simulink model "kurtosis"  (R2012b)
settings: Solver=ode45  StartTime=0.0  StopTime=3171  RelTol=1e-3
libraries: xbsIndex_r4 x3174, casper_library_flow_control x64, casper_library_misc x1, simulink_xsg_bridge x1
(part 3 of 24)

== system kurtosis/kurtosis/kurtosis_origin_moments_2 ==
  sync_in : Inport
  x_in : Inport  Port=2
  abs_x_sq : Subsystem
  abs_x_sq_del : xbsIndex_r4/Delay  rst=off  infoeditControl=Selection of Reset will increase slice count due to use of real FFs and instead of SRLs  en=off  latency=5  dbl_ovrd=off  reg_retiming=off  block_type=delay
  c_to_ri_xin : Subsystem
  cplx_sq : Subsystem
  ri_to_c_x_3rd : Subsystem
  square_real : xbsIndex_r4/Mult  precision=Full  arith_type="Signed  (2's comp)"  n_bits=36  bin_pt=34  quantization=Truncate  overflow=Wrap  en=off  latency=5  dbl_ovrd=off  use_behavioral_HDL=off  opt=Speed  use_embedded=on  optimum_pipeline=off  pipeline=on  use_rpm=on  placement_style=Triangular  block_type=mult
  sync_delay : xbsIndex_r4/Delay  rst=off  infoeditControl=Selection of Reset will increase slice count due to use of real FFs and instead of SRLs  en=off  latency=10  dbl_ovrd=off  reg_retiming=off  block_type=delay
  third_power_im : xbsIndex_r4/Mult  precision=Full  arith_type="Signed  (2's comp)"  n_bits=36  bin_pt=34  quantization=Truncate  overflow=Wrap  en=off  latency=5  dbl_ovrd=off  use_behavioral_HDL=off  opt=Speed  use_embedded=on  optimum_pipeline=off  pipeline=on  use_rpm=on  placement_style=Triangular  block_type=mult
  third_power_re : xbsIndex_r4/Mult  precision=Full  arith_type="Signed  (2's comp)"  n_bits=36  bin_pt=34  quantization=Truncate  overflow=Wrap  en=off  latency=5  dbl_ovrd=off  use_behavioral_HDL=off  opt=Speed  use_embedded=on  optimum_pipeline=off  pipeline=on  use_rpm=on  placement_style=Triangular  block_type=mult
  x_delay : xbsIndex_r4/Delay  rst=off  infoeditControl=Selection of Reset will increase slice count due to use of real FFs and instead of SRLs  en=off  latency=10  dbl_ovrd=off  reg_retiming=off  block_type=delay
  x_im_del : xbsIndex_r4/Delay  rst=off  infoeditControl=Selection of Reset will increase slice count due to use of real FFs and instead of SRLs  en=off  latency=5  dbl_ovrd=off  reg_retiming=off  block_type=delay
  x_re_del : xbsIndex_r4/Delay  rst=off  infoeditControl=Selection of Reset will increase slice count due to use of real FFs and instead of SRLs  en=off  latency=5  dbl_ovrd=off  reg_retiming=off  block_type=delay
  x_sq_del : xbsIndex_r4/Delay  rst=off  infoeditControl=Selection of Reset will increase slice count due to use of real FFs and instead of SRLs  en=off  latency=4  dbl_ovrd=off  reg_retiming=off  block_type=delay
  sync_out : Outport
  x : Outport  Port=2
  x^2 : Outport  Port=3
  |x|^2 : Outport  Port=4
  |x|^4 : Outport  Port=5
  x|x|^2 : Outport  Port=6
  wires:
  x_in/1 -> c_to_ri_xin/1(c), abs_x_sq/1(c), cplx_sq/2(b), cplx_sq/1(a), x_delay/1
  abs_x_sq/1(power) -> third_power_im/2, third_power_re/2, square_real/2, square_real/1, abs_x_sq_del/1
  ri_to_c_x_3rd/1(c) -> x|x|^2/1
  third_power_im/1 -> ri_to_c_x_3rd/2(im)
  third_power_re/1 -> ri_to_c_x_3rd/1(re)
  x_im_del/1 -> third_power_im/1
  x_re_del/1 -> third_power_re/1
  c_to_ri_xin/2(im) -> x_im_del/1
  c_to_ri_xin/1(re) -> x_re_del/1
  square_real/1 -> |x|^4/1
  abs_x_sq_del/1 -> |x|^2/1
  x_sq_del/1 -> x^2/1
  cplx_sq/1(c) -> x_sq_del/1
  x_delay/1 -> x/1
  sync_delay/1 -> sync_out/1
  sync_in/1 -> sync_delay/1

== system kurtosis/kurtosis/kurtosis_origin_moments_3 ==
  sync_in : Inport
  x_in : Inport  Port=2
  abs_x_sq : Subsystem
  abs_x_sq_del : xbsIndex_r4/Delay  rst=off  infoeditControl=Selection of Reset will increase slice count due to use of real FFs and instead of SRLs  en=off  latency=5  dbl_ovrd=off  reg_retiming=off  block_type=delay
  c_to_ri_xin : Subsystem
  cplx_sq : Subsystem
  ri_to_c_x_3rd : Subsystem
  square_real : xbsIndex_r4/Mult  precision=Full  arith_type="Signed  (2's comp)"  n_bits=36  bin_pt=34  quantization=Truncate  overflow=Wrap  en=off  latency=5  dbl_ovrd=off  use_behavioral_HDL=off  opt=Speed  use_embedded=on  optimum_pipeline=off  pipeline=on  use_rpm=on  placement_style=Triangular  block_type=mult
  sync_delay : xbsIndex_r4/Delay  rst=off  infoeditControl=Selection of Reset will increase slice count due to use of real FFs and instead of SRLs  en=off  latency=10  dbl_ovrd=off  reg_retiming=off  block_type=delay
  third_power_im : xbsIndex_r4/Mult  precision=Full  arith_type="Signed  (2's comp)"  n_bits=36  bin_pt=34  quantization=Truncate  overflow=Wrap  en=off  latency=5  dbl_ovrd=off  use_behavioral_HDL=off  opt=Speed  use_embedded=on  optimum_pipeline=off  pipeline=on  use_rpm=on  placement_style=Triangular  block_type=mult
  third_power_re : xbsIndex_r4/Mult  precision=Full  arith_type="Signed  (2's comp)"  n_bits=36  bin_pt=34  quantization=Truncate  overflow=Wrap  en=off  latency=5  dbl_ovrd=off  use_behavioral_HDL=off  opt=Speed  use_embedded=on  optimum_pipeline=off  pipeline=on  use_rpm=on  placement_style=Triangular  block_type=mult
  x_delay : xbsIndex_r4/Delay  rst=off  infoeditControl=Selection of Reset will increase slice count due to use of real FFs and instead of SRLs  en=off  latency=10  dbl_ovrd=off  reg_retiming=off  block_type=delay
  x_im_del : xbsIndex_r4/Delay  rst=off  infoeditControl=Selection of Reset will increase slice count due to use of real FFs and instead of SRLs  en=off  latency=5  dbl_ovrd=off  reg_retiming=off  block_type=delay
  x_re_del : xbsIndex_r4/Delay  rst=off  infoeditControl=Selection of Reset will increase slice count due to use of real FFs and instead of SRLs  en=off  latency=5  dbl_ovrd=off  reg_retiming=off  block_type=delay
  x_sq_del : xbsIndex_r4/Delay  rst=off  infoeditControl=Selection of Reset will increase slice count due to use of real FFs and instead of SRLs  en=off  latency=4  dbl_ovrd=off  reg_retiming=off  block_type=delay
  sync_out : Outport
  x : Outport  Port=2
  x^2 : Outport  Port=3
  |x|^2 : Outport  Port=4
  |x|^4 : Outport  Port=5
  x|x|^2 : Outport  Port=6
  wires:
  x_in/1 -> c_to_ri_xin/1(c), abs_x_sq/1(c), cplx_sq/2(b), cplx_sq/1(a), x_delay/1
  abs_x_sq/1(power) -> third_power_im/2, third_power_re/2, square_real/2, square_real/1, abs_x_sq_del/1
  ri_to_c_x_3rd/1(c) -> x|x|^2/1
  third_power_im/1 -> ri_to_c_x_3rd/2(im)
  third_power_re/1 -> ri_to_c_x_3rd/1(re)
  x_im_del/1 -> third_power_im/1
  x_re_del/1 -> third_power_re/1
  c_to_ri_xin/2(im) -> x_im_del/1
  c_to_ri_xin/1(re) -> x_re_del/1
  square_real/1 -> |x|^4/1
  abs_x_sq_del/1 -> |x|^2/1
  x_sq_del/1 -> x^2/1
  cplx_sq/1(c) -> x_sq_del/1
  x_delay/1 -> x/1
  sync_delay/1 -> sync_out/1
  sync_in/1 -> sync_delay/1

== system kurtosis/kurtosis/kurtosis_origin_moments_4 ==
  sync_in : Inport
  x_in : Inport  Port=2
  abs_x_sq : Subsystem
  abs_x_sq_del : xbsIndex_r4/Delay  rst=off  infoeditControl=Selection of Reset will increase slice count due to use of real FFs and instead of SRLs  en=off  latency=5  dbl_ovrd=off  reg_retiming=off  block_type=delay
  c_to_ri_xin : Subsystem
  cplx_sq : Subsystem
  ri_to_c_x_3rd : Subsystem
  square_real : xbsIndex_r4/Mult  precision=Full  arith_type="Signed  (2's comp)"  n_bits=36  bin_pt=34  quantization=Truncate  overflow=Wrap  en=off  latency=5  dbl_ovrd=off  use_behavioral_HDL=off  opt=Speed  use_embedded=on  optimum_pipeline=off  pipeline=on  use_rpm=on  placement_style=Triangular  block_type=mult
  sync_delay : xbsIndex_r4/Delay  rst=off  infoeditControl=Selection of Reset will increase slice count due to use of real FFs and instead of SRLs  en=off  latency=10  dbl_ovrd=off  reg_retiming=off  block_type=delay
  third_power_im : xbsIndex_r4/Mult  precision=Full  arith_type="Signed  (2's comp)"  n_bits=36  bin_pt=34  quantization=Truncate  overflow=Wrap  en=off  latency=5  dbl_ovrd=off  use_behavioral_HDL=off  opt=Speed  use_embedded=on  optimum_pipeline=off  pipeline=on  use_rpm=on  placement_style=Triangular  block_type=mult
  third_power_re : xbsIndex_r4/Mult  precision=Full  arith_type="Signed  (2's comp)"  n_bits=36  bin_pt=34  quantization=Truncate  overflow=Wrap  en=off  latency=5  dbl_ovrd=off  use_behavioral_HDL=off  opt=Speed  use_embedded=on  optimum_pipeline=off  pipeline=on  use_rpm=on  placement_style=Triangular  block_type=mult
  x_delay : xbsIndex_r4/Delay  rst=off  infoeditControl=Selection of Reset will increase slice count due to use of real FFs and instead of SRLs  en=off  latency=10  dbl_ovrd=off  reg_retiming=off  block_type=delay
  x_im_del : xbsIndex_r4/Delay  rst=off  infoeditControl=Selection of Reset will increase slice count due to use of real FFs and instead of SRLs  en=off  latency=5  dbl_ovrd=off  reg_retiming=off  block_type=delay
  x_re_del : xbsIndex_r4/Delay  rst=off  infoeditControl=Selection of Reset will increase slice count due to use of real FFs and instead of SRLs  en=off  latency=5  dbl_ovrd=off  reg_retiming=off  block_type=delay
  x_sq_del : xbsIndex_r4/Delay  rst=off  infoeditControl=Selection of Reset will increase slice count due to use of real FFs and instead of SRLs  en=off  latency=4  dbl_ovrd=off  reg_retiming=off  block_type=delay
  sync_out : Outport
  x : Outport  Port=2
  x^2 : Outport  Port=3
  |x|^2 : Outport  Port=4
  |x|^4 : Outport  Port=5
  x|x|^2 : Outport  Port=6
  wires:
  x_in/1 -> c_to_ri_xin/1(c), abs_x_sq/1(c), cplx_sq/2(b), cplx_sq/1(a), x_delay/1
  abs_x_sq/1(power) -> third_power_im/2, third_power_re/2, square_real/2, square_real/1, abs_x_sq_del/1
  ri_to_c_x_3rd/1(c) -> x|x|^2/1
  third_power_im/1 -> ri_to_c_x_3rd/2(im)
  third_power_re/1 -> ri_to_c_x_3rd/1(re)
  x_im_del/1 -> third_power_im/1
  x_re_del/1 -> third_power_re/1
  c_to_ri_xin/2(im) -> x_im_del/1
  c_to_ri_xin/1(re) -> x_re_del/1
  square_real/1 -> |x|^4/1
  abs_x_sq_del/1 -> |x|^2/1
  x_sq_del/1 -> x^2/1
  cplx_sq/1(c) -> x_sq_del/1
  x_delay/1 -> x/1
  sync_delay/1 -> sync_out/1
  sync_in/1 -> sync_delay/1

== system kurtosis/kurtosis/kurtosis_origin_moments_5 ==
  sync_in : Inport
  x_in : Inport  Port=2
  abs_x_sq : Subsystem
  abs_x_sq_del : xbsIndex_r4/Delay  rst=off  infoeditControl=Selection of Reset will increase slice count due to use of real FFs and instead of SRLs  en=off  latency=5  dbl_ovrd=off  reg_retiming=off  block_type=delay
  c_to_ri_xin : Subsystem
  cplx_sq : Subsystem
  ri_to_c_x_3rd : Subsystem
  square_real : xbsIndex_r4/Mult  precision=Full  arith_type="Signed  (2's comp)"  n_bits=36  bin_pt=34  quantization=Truncate  overflow=Wrap  en=off  latency=5  dbl_ovrd=off  use_behavioral_HDL=off  opt=Speed  use_embedded=on  optimum_pipeline=off  pipeline=on  use_rpm=on  placement_style=Triangular  block_type=mult
  sync_delay : xbsIndex_r4/Delay  rst=off  infoeditControl=Selection of Reset will increase slice count due to use of real FFs and instead of SRLs  en=off  latency=10  dbl_ovrd=off  reg_retiming=off  block_type=delay
  third_power_im : xbsIndex_r4/Mult  precision=Full  arith_type="Signed  (2's comp)"  n_bits=36  bin_pt=34  quantization=Truncate  overflow=Wrap  en=off  latency=5  dbl_ovrd=off  use_behavioral_HDL=off  opt=Speed  use_embedded=on  optimum_pipeline=off  pipeline=on  use_rpm=on  placement_style=Triangular  block_type=mult
  third_power_re : xbsIndex_r4/Mult  precision=Full  arith_type="Signed  (2's comp)"  n_bits=36  bin_pt=34  quantization=Truncate  overflow=Wrap  en=off  latency=5  dbl_ovrd=off  use_behavioral_HDL=off  opt=Speed  use_embedded=on  optimum_pipeline=off  pipeline=on  use_rpm=on  placement_style=Triangular  block_type=mult
  x_delay : xbsIndex_r4/Delay  rst=off  infoeditControl=Selection of Reset will increase slice count due to use of real FFs and instead of SRLs  en=off  latency=10  dbl_ovrd=off  reg_retiming=off  block_type=delay
  x_im_del : xbsIndex_r4/Delay  rst=off  infoeditControl=Selection of Reset will increase slice count due to use of real FFs and instead of SRLs  en=off  latency=5  dbl_ovrd=off  reg_retiming=off  block_type=delay
  x_re_del : xbsIndex_r4/Delay  rst=off  infoeditControl=Selection of Reset will increase slice count due to use of real FFs and instead of SRLs  en=off  latency=5  dbl_ovrd=off  reg_retiming=off  block_type=delay
  x_sq_del : xbsIndex_r4/Delay  rst=off  infoeditControl=Selection of Reset will increase slice count due to use of real FFs and instead of SRLs  en=off  latency=4  dbl_ovrd=off  reg_retiming=off  block_type=delay
  sync_out : Outport
  x : Outport  Port=2
  x^2 : Outport  Port=3
  |x|^2 : Outport  Port=4
  |x|^4 : Outport  Port=5
  x|x|^2 : Outport  Port=6
  wires:
  x_in/1 -> c_to_ri_xin/1(c), abs_x_sq/1(c), cplx_sq/2(b), cplx_sq/1(a), x_delay/1
  abs_x_sq/1(power) -> third_power_im/2, third_power_re/2, square_real/2, square_real/1, abs_x_sq_del/1
  ri_to_c_x_3rd/1(c) -> x|x|^2/1
  third_power_im/1 -> ri_to_c_x_3rd/2(im)
  third_power_re/1 -> ri_to_c_x_3rd/1(re)
  x_im_del/1 -> third_power_im/1
  x_re_del/1 -> third_power_re/1
  c_to_ri_xin/2(im) -> x_im_del/1
  c_to_ri_xin/1(re) -> x_re_del/1
  square_real/1 -> |x|^4/1
  abs_x_sq_del/1 -> |x|^2/1
  x_sq_del/1 -> x^2/1
  cplx_sq/1(c) -> x_sq_del/1
  x_delay/1 -> x/1
  sync_delay/1 -> sync_out/1
  sync_in/1 -> sync_delay/1

== system kurtosis/kurtosis/kurtosis_origin_moments_6 ==
  sync_in : Inport
  x_in : Inport  Port=2
  abs_x_sq : Subsystem
  abs_x_sq_del : xbsIndex_r4/Delay  rst=off  infoeditControl=Selection of Reset will increase slice count due to use of real FFs and instead of SRLs  en=off  latency=5  dbl_ovrd=off  reg_retiming=off  block_type=delay
  c_to_ri_xin : Subsystem
  cplx_sq : Subsystem
  ri_to_c_x_3rd : Subsystem
  square_real : xbsIndex_r4/Mult  precision=Full  arith_type="Signed  (2's comp)"  n_bits=36  bin_pt=34  quantization=Truncate  overflow=Wrap  en=off  latency=5  dbl_ovrd=off  use_behavioral_HDL=off  opt=Speed  use_embedded=on  optimum_pipeline=off  pipeline=on  use_rpm=on  placement_style=Triangular  block_type=mult
  sync_delay : xbsIndex_r4/Delay  rst=off  infoeditControl=Selection of Reset will increase slice count due to use of real FFs and instead of SRLs  en=off  latency=10  dbl_ovrd=off  reg_retiming=off  block_type=delay
  third_power_im : xbsIndex_r4/Mult  precision=Full  arith_type="Signed  (2's comp)"  n_bits=36  bin_pt=34  quantization=Truncate  overflow=Wrap  en=off  latency=5  dbl_ovrd=off  use_behavioral_HDL=off  opt=Speed  use_embedded=on  optimum_pipeline=off  pipeline=on  use_rpm=on  placement_style=Triangular  block_type=mult
  third_power_re : xbsIndex_r4/Mult  precision=Full  arith_type="Signed  (2's comp)"  n_bits=36  bin_pt=34  quantization=Truncate  overflow=Wrap  en=off  latency=5  dbl_ovrd=off  use_behavioral_HDL=off  opt=Speed  use_embedded=on  optimum_pipeline=off  pipeline=on  use_rpm=on  placement_style=Triangular  block_type=mult
  x_delay : xbsIndex_r4/Delay  rst=off  infoeditControl=Selection of Reset will increase slice count due to use of real FFs and instead of SRLs  en=off  latency=10  dbl_ovrd=off  reg_retiming=off  block_type=delay
  x_im_del : xbsIndex_r4/Delay  rst=off  infoeditControl=Selection of Reset will increase slice count due to use of real FFs and instead of SRLs  en=off  latency=5  dbl_ovrd=off  reg_retiming=off  block_type=delay
  x_re_del : xbsIndex_r4/Delay  rst=off  infoeditControl=Selection of Reset will increase slice count due to use of real FFs and instead of SRLs  en=off  latency=5  dbl_ovrd=off  reg_retiming=off  block_type=delay
  x_sq_del : xbsIndex_r4/Delay  rst=off  infoeditControl=Selection of Reset will increase slice count due to use of real FFs and instead of SRLs  en=off  latency=4  dbl_ovrd=off  reg_retiming=off  block_type=delay
  sync_out : Outport
  x : Outport  Port=2
  x^2 : Outport  Port=3
  |x|^2 : Outport  Port=4
  |x|^4 : Outport  Port=5
  x|x|^2 : Outport  Port=6
  wires:
  x_in/1 -> c_to_ri_xin/1(c), abs_x_sq/1(c), cplx_sq/2(b), cplx_sq/1(a), x_delay/1
  abs_x_sq/1(power) -> third_power_im/2, third_power_re/2, square_real/2, square_real/1, abs_x_sq_del/1
  ri_to_c_x_3rd/1(c) -> x|x|^2/1
  third_power_im/1 -> ri_to_c_x_3rd/2(im)
  third_power_re/1 -> ri_to_c_x_3rd/1(re)
  x_im_del/1 -> third_power_im/1
  x_re_del/1 -> third_power_re/1
  c_to_ri_xin/2(im) -> x_im_del/1
  c_to_ri_xin/1(re) -> x_re_del/1
  square_real/1 -> |x|^4/1
  abs_x_sq_del/1 -> |x|^2/1
  x_sq_del/1 -> x^2/1
  cplx_sq/1(c) -> x_sq_del/1
  x_delay/1 -> x/1
  sync_delay/1 -> sync_out/1
  sync_in/1 -> sync_delay/1

== system kurtosis/kurtosis/kurtosis_origin_moments_7 ==
  sync_in : Inport
  x_in : Inport  Port=2
  abs_x_sq : Subsystem
  abs_x_sq_del : xbsIndex_r4/Delay  rst=off  infoeditControl=Selection of Reset will increase slice count due to use of real FFs and instead of SRLs  en=off  latency=5  dbl_ovrd=off  reg_retiming=off  block_type=delay
  c_to_ri_xin : Subsystem
  cplx_sq : Subsystem
  ri_to_c_x_3rd : Subsystem
  square_real : xbsIndex_r4/Mult  precision=Full  arith_type="Signed  (2's comp)"  n_bits=36  bin_pt=34  quantization=Truncate  overflow=Wrap  en=off  latency=5  dbl_ovrd=off  use_behavioral_HDL=off  opt=Speed  use_embedded=on  optimum_pipeline=off  pipeline=on  use_rpm=on  placement_style=Triangular  block_type=mult
  sync_delay : xbsIndex_r4/Delay  rst=off  infoeditControl=Selection of Reset will increase slice count due to use of real FFs and instead of SRLs  en=off  latency=10  dbl_ovrd=off  reg_retiming=off  block_type=delay
  third_power_im : xbsIndex_r4/Mult  precision=Full  arith_type="Signed  (2's comp)"  n_bits=36  bin_pt=34  quantization=Truncate  overflow=Wrap  en=off  latency=5  dbl_ovrd=off  use_behavioral_HDL=off  opt=Speed  use_embedded=on  optimum_pipeline=off  pipeline=on  use_rpm=on  placement_style=Triangular  block_type=mult
  third_power_re : xbsIndex_r4/Mult  precision=Full  arith_type="Signed  (2's comp)"  n_bits=36  bin_pt=34  quantization=Truncate  overflow=Wrap  en=off  latency=5  dbl_ovrd=off  use_behavioral_HDL=off  opt=Speed  use_embedded=on  optimum_pipeline=off  pipeline=on  use_rpm=on  placement_style=Triangular  block_type=mult
  x_delay : xbsIndex_r4/Delay  rst=off  infoeditControl=Selection of Reset will increase slice count due to use of real FFs and instead of SRLs  en=off  latency=10  dbl_ovrd=off  reg_retiming=off  block_type=delay
  x_im_del : xbsIndex_r4/Delay  rst=off  infoeditControl=Selection of Reset will increase slice count due to use of real FFs and instead of SRLs  en=off  latency=5  dbl_ovrd=off  reg_retiming=off  block_type=delay
  x_re_del : xbsIndex_r4/Delay  rst=off  infoeditControl=Selection of Reset will increase slice count due to use of real FFs and instead of SRLs  en=off  latency=5  dbl_ovrd=off  reg_retiming=off  block_type=delay
  x_sq_del : xbsIndex_r4/Delay  rst=off  infoeditControl=Selection of Reset will increase slice count due to use of real FFs and instead of SRLs  en=off  latency=4  dbl_ovrd=off  reg_retiming=off  block_type=delay
  sync_out : Outport
  x : Outport  Port=2
  x^2 : Outport  Port=3
  |x|^2 : Outport  Port=4
  |x|^4 : Outport  Port=5
  x|x|^2 : Outport  Port=6
  wires:
  x_in/1 -> c_to_ri_xin/1(c), abs_x_sq/1(c), cplx_sq/2(b), cplx_sq/1(a), x_delay/1
  abs_x_sq/1(power) -> third_power_im/2, third_power_re/2, square_real/2, square_real/1, abs_x_sq_del/1
  ri_to_c_x_3rd/1(c) -> x|x|^2/1
  third_power_im/1 -> ri_to_c_x_3rd/2(im)
  third_power_re/1 -> ri_to_c_x_3rd/1(re)
  x_im_del/1 -> third_power_im/1
  x_re_del/1 -> third_power_re/1
  c_to_ri_xin/2(im) -> x_im_del/1
  c_to_ri_xin/1(re) -> x_re_del/1
  square_real/1 -> |x|^4/1
  abs_x_sq_del/1 -> |x|^2/1
  x_sq_del/1 -> x^2/1
  cplx_sq/1(c) -> x_sq_del/1
  x_delay/1 -> x/1
  sync_delay/1 -> sync_out/1
  sync_in/1 -> sync_delay/1

== system kurtosis/kurtosis/kurtosis_origin_moments_8 ==
  sync_in : Inport
  x_in : Inport  Port=2
  abs_x_sq : Subsystem
  abs_x_sq_del : xbsIndex_r4/Delay  rst=off  infoeditControl=Selection of Reset will increase slice count due to use of real FFs and instead of SRLs  en=off  latency=5  dbl_ovrd=off  reg_retiming=off  block_type=delay
  c_to_ri_xin : Subsystem
  cplx_sq : Subsystem
  ri_to_c_x_3rd : Subsystem
  square_real : xbsIndex_r4/Mult  precision=Full  arith_type="Signed  (2's comp)"  n_bits=36  bin_pt=34  quantization=Truncate  overflow=Wrap  en=off  latency=5  dbl_ovrd=off  use_behavioral_HDL=off  opt=Speed  use_embedded=on  optimum_pipeline=off  pipeline=on  use_rpm=on  placement_style=Triangular  block_type=mult
  sync_delay : xbsIndex_r4/Delay  rst=off  infoeditControl=Selection of Reset will increase slice count due to use of real FFs and instead of SRLs  en=off  latency=10  dbl_ovrd=off  reg_retiming=off  block_type=delay
  third_power_im : xbsIndex_r4/Mult  precision=Full  arith_type="Signed  (2's comp)"  n_bits=36  bin_pt=34  quantization=Truncate  overflow=Wrap  en=off  latency=5  dbl_ovrd=off  use_behavioral_HDL=off  opt=Speed  use_embedded=on  optimum_pipeline=off  pipeline=on  use_rpm=on  placement_style=Triangular  block_type=mult
  third_power_re : xbsIndex_r4/Mult  precision=Full  arith_type="Signed  (2's comp)"  n_bits=36  bin_pt=34  quantization=Truncate  overflow=Wrap  en=off  latency=5  dbl_ovrd=off  use_behavioral_HDL=off  opt=Speed  use_embedded=on  optimum_pipeline=off  pipeline=on  use_rpm=on  placement_style=Triangular  block_type=mult
  x_delay : xbsIndex_r4/Delay  rst=off  infoeditControl=Selection of Reset will increase slice count due to use of real FFs and instead of SRLs  en=off  latency=10  dbl_ovrd=off  reg_retiming=off  block_type=delay
  x_im_del : xbsIndex_r4/Delay  rst=off  infoeditControl=Selection of Reset will increase slice count due to use of real FFs and instead of SRLs  en=off  latency=5  dbl_ovrd=off  reg_retiming=off  block_type=delay
  x_re_del : xbsIndex_r4/Delay  rst=off  infoeditControl=Selection of Reset will increase slice count due to use of real FFs and instead of SRLs  en=off  latency=5  dbl_ovrd=off  reg_retiming=off  block_type=delay
  x_sq_del : xbsIndex_r4/Delay  rst=off  infoeditControl=Selection of Reset will increase slice count due to use of real FFs and instead of SRLs  en=off  latency=4  dbl_ovrd=off  reg_retiming=off  block_type=delay
  sync_out : Outport
  x : Outport  Port=2
  x^2 : Outport  Port=3
  |x|^2 : Outport  Port=4
  |x|^4 : Outport  Port=5
  x|x|^2 : Outport  Port=6
  wires:
  x_in/1 -> c_to_ri_xin/1(c), abs_x_sq/1(c), cplx_sq/2(b), cplx_sq/1(a), x_delay/1
  abs_x_sq/1(power) -> third_power_im/2, third_power_re/2, square_real/2, square_real/1, abs_x_sq_del/1
  ri_to_c_x_3rd/1(c) -> x|x|^2/1
  third_power_im/1 -> ri_to_c_x_3rd/2(im)
  third_power_re/1 -> ri_to_c_x_3rd/1(re)
  x_im_del/1 -> third_power_im/1
  x_re_del/1 -> third_power_re/1
  c_to_ri_xin/2(im) -> x_im_del/1
  c_to_ri_xin/1(re) -> x_re_del/1
  square_real/1 -> |x|^4/1
  abs_x_sq_del/1 -> |x|^2/1
  x_sq_del/1 -> x^2/1
  cplx_sq/1(c) -> x_sq_del/1
  x_delay/1 -> x/1
  sync_delay/1 -> sync_out/1
  sync_in/1 -> sync_delay/1

== system kurtosis/kurtosis/m_x_im_ser ==
  load : Inport
  din_1 : Inport  Port=2
  din_2 : Inport  Port=3
  din_3 : Inport  Port=4
  din_4 : Inport  Port=5
  din_5 : Inport  Port=6
  din_6 : Inport  Port=7
  din_7 : Inport  Port=8
  din_8 : Inport  Port=9
  addr_counter : xbsIndex_r4/Counter  cnt_type=Free Running  cnt_to=Inf  operation=Up  start_count=0  cnt_by_val=1  arith_type=Unsigned  n_bits=4  bin_pt=0  load_pin=off  rst=on  en=off  explicit_period=on  period=1  dbl_ovrd=off  use_behavioral_HDL=off  implementation=Fabric  block_type=counter
  addr_del : xbsIndex_r4/Delay  rst=off  infoeditControl=Selection of Reset will increase slice count due to use of real FFs and instead of SRLs  en=off  latency=1  dbl_ovrd=off  reg_retiming=off  block_type=delay
  par_to_ser : Subsystem  AncestorBlock=casper_library_flow_control/parallel_to_serial_converter  mask(parallel_to_serial_converter){pin_width=200, sout_width=25}
      mask prompts: pin_width "Parallel Input Width"; sout_width "Serial Output Width"
      mask help:
      | This block takes as input a parallel bus of specified width.
      | When the load signal 'ld' is asserted, this data is broken into
      | pieces of width specified by the serial output width and
      | stored into different registers chained to form a shift register.
      | If the 'shift' input is subsequently asserted, the shift register
      | returns as output a new piece of data of width sout_width.  This data
      | is the next least significant piece of the original bus.  The converter
      | serializes SMALL ENDIAN.
      |
      | Note that the load operation automatically loads the least significant
      | bits into the register closest to the output, so the first 'shift'
      | assertion changes the data output from bits [sout_width-1:0] to
      | bits [2*sout_width-1:sout_width].
      mask init:
      | parallel_to_serial_converter_init(gcb, ...
      |     'pin_width', pin_width, ...
      |     'sout_width', sout_width);
  pin_concat : Subsystem
  pulse_ext : Subsystem
  reinterp : xbsIndex_r4/Reinterpret  force_arith_type=on  arith_type="Signed  (2's comp)"  force_bin_pt=on  bin_pt=24  block_type=reinterpret
  addr : Outport
  ser_data : Outport  Port=2
  valid : Outport  Port=3
  wires:
  load/1 -> addr_counter/1, par_to_ser/2(ld), pulse_ext/1(ld)
  pulse_ext/1(shift) -> par_to_ser/3(shift), valid/1  "shift"
  addr_del/1 -> addr/1
  addr_counter/1 -> addr_del/1
  reinterp/1 -> ser_data/1
  par_to_ser/1(sout) -> reinterp/1  "sout"
  pin_concat/1(out) -> par_to_ser/1(pin)
  din_8/1 -> pin_concat/8(in7)
  din_7/1 -> pin_concat/7(in6)
  din_6/1 -> pin_concat/6(in5)
  din_5/1 -> pin_concat/5(in4)
  din_4/1 -> pin_concat/4(in3)
  din_3/1 -> pin_concat/3(in2)
  din_2/1 -> pin_concat/2(in1)
  din_1/1 -> pin_concat/1(in0)

== system kurtosis/kurtosis/m_x_re_ser ==
  load : Inport
  din_1 : Inport  Port=2
  din_2 : Inport  Port=3
  din_3 : Inport  Port=4
  din_4 : Inport  Port=5
  din_5 : Inport  Port=6
  din_6 : Inport  Port=7
  din_7 : Inport  Port=8
  din_8 : Inport  Port=9
  addr_counter : xbsIndex_r4/Counter  cnt_type=Free Running  cnt_to=Inf  operation=Up  start_count=0  cnt_by_val=1  arith_type=Unsigned  n_bits=4  bin_pt=0  load_pin=off  rst=on  en=off  explicit_period=on  period=1  dbl_ovrd=off  use_behavioral_HDL=off  implementation=Fabric  block_type=counter
  addr_del : xbsIndex_r4/Delay  rst=off  infoeditControl=Selection of Reset will increase slice count due to use of real FFs and instead of SRLs  en=off  latency=1  dbl_ovrd=off  reg_retiming=off  block_type=delay
  par_to_ser : Subsystem  AncestorBlock=casper_library_flow_control/parallel_to_serial_converter  mask(parallel_to_serial_converter){pin_width=200, sout_width=25}
      mask prompts: pin_width "Parallel Input Width"; sout_width "Serial Output Width"
      mask help:
      | This block takes as input a parallel bus of specified width.
      | When the load signal 'ld' is asserted, this data is broken into
      | pieces of width specified by the serial output width and
      | stored into different registers chained to form a shift register.
      | If the 'shift' input is subsequently asserted, the shift register
      | returns as output a new piece of data of width sout_width.  This data
      | is the next least significant piece of the original bus.  The converter
      | serializes SMALL ENDIAN.
      |
      | Note that the load operation automatically loads the least significant
      | bits into the register closest to the output, so the first 'shift'
      | assertion changes the data output from bits [sout_width-1:0] to
      | bits [2*sout_width-1:sout_width].
      mask init:
      | parallel_to_serial_converter_init(gcb, ...
      |     'pin_width', pin_width, ...
      |     'sout_width', sout_width);
  pin_concat : Subsystem
  pulse_ext : Subsystem
  reinterp : xbsIndex_r4/Reinterpret  force_arith_type=on  arith_type="Signed  (2's comp)"  force_bin_pt=on  bin_pt=24  block_type=reinterpret
  addr : Outport
  ser_data : Outport  Port=2
  valid : Outport  Port=3
  wires:
  load/1 -> addr_counter/1, par_to_ser/2(ld), pulse_ext/1(ld)
  pulse_ext/1(shift) -> par_to_ser/3(shift), valid/1  "shift"
  addr_del/1 -> addr/1
  addr_counter/1 -> addr_del/1
  reinterp/1 -> ser_data/1
  par_to_ser/1(sout) -> reinterp/1  "sout"
  pin_concat/1(out) -> par_to_ser/1(pin)
  din_8/1 -> pin_concat/8(in7)
  din_7/1 -> pin_concat/7(in6)
  din_6/1 -> pin_concat/6(in5)
  din_5/1 -> pin_concat/5(in4)
  din_4/1 -> pin_concat/4(in3)
  din_3/1 -> pin_concat/3(in2)
  din_2/1 -> pin_concat/2(in1)
  din_1/1 -> pin_concat/1(in0)

== system kurtosis/kurtosis/x_3rd_im_ser ==
  load : Inport
  din_1 : Inport  Port=2
  din_2 : Inport  Port=3
  din_3 : Inport  Port=4
  din_4 : Inport  Port=5
  din_5 : Inport  Port=6
  din_6 : Inport  Port=7
  din_7 : Inport  Port=8
  din_8 : Inport  Port=9
  addr_counter : xbsIndex_r4/Counter  cnt_type=Free Running  cnt_to=Inf  operation=Up  start_count=0  cnt_by_val=1  arith_type=Unsigned  n_bits=4  bin_pt=0  load_pin=off  rst=on  en=off  explicit_period=on  period=1  dbl_ovrd=off  use_behavioral_HDL=off  implementation=Fabric  block_type=counter
  addr_del : xbsIndex_r4/Delay  rst=off  infoeditControl=Selection of Reset will increase slice count due to use of real FFs and instead of SRLs  en=off  latency=1  dbl_ovrd=off  reg_retiming=off  block_type=delay
  par_to_ser : Subsystem  AncestorBlock=casper_library_flow_control/parallel_to_serial_converter  mask(parallel_to_serial_converter){pin_width=280, sout_width=35}
      mask prompts: pin_width "Parallel Input Width"; sout_width "Serial Output Width"
      mask help:
      | This block takes as input a parallel bus of specified width.
      | When the load signal 'ld' is asserted, this data is broken into
      | pieces of width specified by the serial output width and
      | stored into different registers chained to form a shift register.
      | If the 'shift' input is subsequently asserted, the shift register
      | returns as output a new piece of data of width sout_width.  This data
      | is the next least significant piece of the original bus.  The converter
      | serializes SMALL ENDIAN.
      |
      | Note that the load operation automatically loads the least significant
      | bits into the register closest to the output, so the first 'shift'
      | assertion changes the data output from bits [sout_width-1:0] to
      | bits [2*sout_width-1:sout_width].
      mask init:
      | parallel_to_serial_converter_init(gcb, ...
      |     'pin_width', pin_width, ...
      |     'sout_width', sout_width);
  pin_concat : Subsystem
  pulse_ext : Subsystem
  reinterp : xbsIndex_r4/Reinterpret  force_arith_type=on  arith_type="Signed  (2's comp)"  force_bin_pt=on  bin_pt=22  block_type=reinterpret
  addr : Outport
  ser_data : Outport  Port=2
  valid : Outport  Port=3
  wires:
  load/1 -> addr_counter/1, par_to_ser/2(ld), pulse_ext/1(ld)
  pulse_ext/1(shift) -> par_to_ser/3(shift), valid/1  "shift"
  addr_del/1 -> addr/1
  addr_counter/1 -> addr_del/1
  reinterp/1 -> ser_data/1
  par_to_ser/1(sout) -> reinterp/1  "sout"
  pin_concat/1(out) -> par_to_ser/1(pin)
  din_8/1 -> pin_concat/8(in7)
  din_7/1 -> pin_concat/7(in6)
  din_6/1 -> pin_concat/6(in5)
  din_5/1 -> pin_concat/5(in4)
  din_4/1 -> pin_concat/4(in3)
  din_3/1 -> pin_concat/3(in2)
  din_2/1 -> pin_concat/2(in1)
  din_1/1 -> pin_concat/1(in0)

== system kurtosis/kurtosis/x_3rd_re_ser ==
  load : Inport
  din_1 : Inport  Port=2
  din_2 : Inport  Port=3
  din_3 : Inport  Port=4
  din_4 : Inport  Port=5
  din_5 : Inport  Port=6
  din_6 : Inport  Port=7
  din_7 : Inport  Port=8
  din_8 : Inport  Port=9
  addr_counter : xbsIndex_r4/Counter  cnt_type=Free Running  cnt_to=Inf  operation=Up  start_count=0  cnt_by_val=1  arith_type=Unsigned  n_bits=4  bin_pt=0  load_pin=off  rst=on  en=off  explicit_period=on  period=1  dbl_ovrd=off  use_behavioral_HDL=off  implementation=Fabric  block_type=counter
  addr_del : xbsIndex_r4/Delay  rst=off  infoeditControl=Selection of Reset will increase slice count due to use of real FFs and instead of SRLs  en=off  latency=1  dbl_ovrd=off  reg_retiming=off  block_type=delay
  par_to_ser : Subsystem  AncestorBlock=casper_library_flow_control/parallel_to_serial_converter  mask(parallel_to_serial_converter){pin_width=280, sout_width=35}
      mask prompts: pin_width "Parallel Input Width"; sout_width "Serial Output Width"
      mask help:
      | This block takes as input a parallel bus of specified width.
      | When the load signal 'ld' is asserted, this data is broken into
      | pieces of width specified by the serial output width and
      | stored into different registers chained to form a shift register.
      | If the 'shift' input is subsequently asserted, the shift register
      | returns as output a new piece of data of width sout_width.  This data
      | is the next least significant piece of the original bus.  The converter
      | serializes SMALL ENDIAN.
      |
      | Note that the load operation automatically loads the least significant
      | bits into the register closest to the output, so the first 'shift'
      | assertion changes the data output from bits [sout_width-1:0] to
      | bits [2*sout_width-1:sout_width].
      mask init:
      | parallel_to_serial_converter_init(gcb, ...
      |     'pin_width', pin_width, ...
      |     'sout_width', sout_width);
  pin_concat : Subsystem
  pulse_ext : Subsystem
  reinterp : xbsIndex_r4/Reinterpret  force_arith_type=on  arith_type="Signed  (2's comp)"  force_bin_pt=on  bin_pt=22  block_type=reinterpret
  addr : Outport
  ser_data : Outport  Port=2
  valid : Outport  Port=3
  wires:
  load/1 -> addr_counter/1, par_to_ser/2(ld), pulse_ext/1(ld)
  pulse_ext/1(shift) -> par_to_ser/3(shift), valid/1  "shift"
  addr_del/1 -> addr/1
  addr_counter/1 -> addr_del/1
  reinterp/1 -> ser_data/1
  par_to_ser/1(sout) -> reinterp/1  "sout"
  pin_concat/1(out) -> par_to_ser/1(pin)
  din_8/1 -> pin_concat/8(in7)
  din_7/1 -> pin_concat/7(in6)
  din_6/1 -> pin_concat/6(in5)
  din_5/1 -> pin_concat/5(in4)
  din_4/1 -> pin_concat/4(in3)
  din_3/1 -> pin_concat/3(in2)
  din_2/1 -> pin_concat/2(in1)
  din_1/1 -> pin_concat/1(in0)

== system kurtosis/kurtosis/x_sq_im_ser ==
  load : Inport
  din_1 : Inport  Port=2
  din_2 : Inport  Port=3
  din_3 : Inport  Port=4
  din_4 : Inport  Port=5
  din_5 : Inport  Port=6
  din_6 : Inport  Port=7
  din_7 : Inport  Port=8
  din_8 : Inport  Port=9
  addr_counter : xbsIndex_r4/Counter  cnt_type=Free Running  cnt_to=Inf  operation=Up  start_count=0  cnt_by_val=1  arith_type=Unsigned  n_bits=4  bin_pt=0  load_pin=off  rst=on  en=off  explicit_period=on  period=1  dbl_ovrd=off  use_behavioral_HDL=off  implementation=Fabric  block_type=counter
  addr_del : xbsIndex_r4/Delay  rst=off  infoeditControl=Selection of Reset will increase slice count due to use of real FFs and instead of SRLs  en=off  latency=1  dbl_ovrd=off  reg_retiming=off  block_type=delay
  par_to_ser : Subsystem  AncestorBlock=casper_library_flow_control/parallel_to_serial_converter  mask(parallel_to_serial_converter){pin_width=280, sout_width=35}
      mask prompts: pin_width "Parallel Input Width"; sout_width "Serial Output Width"
      mask help:
      | This block takes as input a parallel bus of specified width.
      | When the load signal 'ld' is asserted, this data is broken into
      | pieces of width specified by the serial output width and
      | stored into different registers chained to form a shift register.
      | If the 'shift' input is subsequently asserted, the shift register
      | returns as output a new piece of data of width sout_width.  This data
      | is the next least significant piece of the original bus.  The converter
      | serializes SMALL ENDIAN.
      |
      | Note that the load operation automatically loads the least significant
      | bits into the register closest to the output, so the first 'shift'
      | assertion changes the data output from bits [sout_width-1:0] to
      | bits [2*sout_width-1:sout_width].
      mask init:
      | parallel_to_serial_converter_init(gcb, ...
      |     'pin_width', pin_width, ...
      |     'sout_width', sout_width);
  pin_concat : Subsystem
  pulse_ext : Subsystem
  reinterp : xbsIndex_r4/Reinterpret  force_arith_type=on  arith_type="Signed  (2's comp)"  force_bin_pt=on  bin_pt=22  block_type=reinterpret
  addr : Outport
  ser_data : Outport  Port=2
  valid : Outport  Port=3
  wires:
  load/1 -> addr_counter/1, par_to_ser/2(ld), pulse_ext/1(ld)
  pulse_ext/1(shift) -> par_to_ser/3(shift), valid/1  "shift"
  addr_del/1 -> addr/1
  addr_counter/1 -> addr_del/1
  reinterp/1 -> ser_data/1
  par_to_ser/1(sout) -> reinterp/1  "sout"
  pin_concat/1(out) -> par_to_ser/1(pin)
  din_8/1 -> pin_concat/8(in7)
  din_7/1 -> pin_concat/7(in6)
  din_6/1 -> pin_concat/6(in5)
  din_5/1 -> pin_concat/5(in4)
  din_4/1 -> pin_concat/4(in3)
  din_3/1 -> pin_concat/3(in2)
  din_2/1 -> pin_concat/2(in1)
  din_1/1 -> pin_concat/1(in0)

== system kurtosis/kurtosis/x_sq_re_ser ==
  load : Inport
  din_1 : Inport  Port=2
  din_2 : Inport  Port=3
  din_3 : Inport  Port=4
  din_4 : Inport  Port=5
  din_5 : Inport  Port=6
  din_6 : Inport  Port=7
  din_7 : Inport  Port=8
  din_8 : Inport  Port=9
  addr_counter : xbsIndex_r4/Counter  cnt_type=Free Running  cnt_to=Inf  operation=Up  start_count=0  cnt_by_val=1  arith_type=Unsigned  n_bits=4  bin_pt=0  load_pin=off  rst=on  en=off  explicit_period=on  period=1  dbl_ovrd=off  use_behavioral_HDL=off  implementation=Fabric  block_type=counter
  addr_del : xbsIndex_r4/Delay  rst=off  infoeditControl=Selection of Reset will increase slice count due to use of real FFs and instead of SRLs  en=off  latency=1  dbl_ovrd=off  reg_retiming=off  block_type=delay
  par_to_ser : Subsystem  AncestorBlock=casper_library_flow_control/parallel_to_serial_converter  mask(parallel_to_serial_converter){pin_width=280, sout_width=35}
      mask prompts: pin_width "Parallel Input Width"; sout_width "Serial Output Width"
      mask help:
      | This block takes as input a parallel bus of specified width.
      | When the load signal 'ld' is asserted, this data is broken into
      | pieces of width specified by the serial output width and
      | stored into different registers chained to form a shift register.
      | If the 'shift' input is subsequently asserted, the shift register
      | returns as output a new piece of data of width sout_width.  This data
      | is the next least significant piece of the original bus.  The converter
      | serializes SMALL ENDIAN.
      |
      | Note that the load operation automatically loads the least significant
      | bits into the register closest to the output, so the first 'shift'
      | assertion changes the data output from bits [sout_width-1:0] to
      | bits [2*sout_width-1:sout_width].
      mask init:
      | parallel_to_serial_converter_init(gcb, ...
      |     'pin_width', pin_width, ...
      |     'sout_width', sout_width);
  pin_concat : Subsystem
  pulse_ext : Subsystem
  reinterp : xbsIndex_r4/Reinterpret  force_arith_type=on  arith_type="Signed  (2's comp)"  force_bin_pt=on  bin_pt=22  block_type=reinterpret
  addr : Outport
  ser_data : Outport  Port=2
  valid : Outport  Port=3
  wires:
  load/1 -> addr_counter/1, par_to_ser/2(ld), pulse_ext/1(ld)
  pulse_ext/1(shift) -> par_to_ser/3(shift), valid/1  "shift"
  addr_del/1 -> addr/1
  addr_counter/1 -> addr_del/1
  reinterp/1 -> ser_data/1
  par_to_ser/1(sout) -> reinterp/1  "sout"
  pin_concat/1(out) -> par_to_ser/1(pin)
  din_8/1 -> pin_concat/8(in7)
  din_7/1 -> pin_concat/7(in6)
  din_6/1 -> pin_concat/6(in5)
  din_5/1 -> pin_concat/5(in4)
  din_4/1 -> pin_concat/4(in3)
  din_3/1 -> pin_concat/3(in2)
  din_2/1 -> pin_concat/2(in1)
  din_1/1 -> pin_concat/1(in0)

== system kurtosis/multi_from_workspace_complex/from_workspace_cplx_1 ==
  c_to_ri_simulink : ComplexToRealImag
  gateway_imag : xbsIndex_r4/Gateway In  gui_display_data_type=Fixed-point  arith_type="Signed  (2's comp)"  n_bits=18  bin_pt=17  preci_type=Single  exp_width=8  frac_width=24  quantization=Truncate  overflow=Wrap  period=1  dbl_ovrd=off  timing_constraint=None  locs_specified=off  LOCs={}  UseAsADC=off  ADCChannel='1'  inherit_from_input=off  hdl_port=on  block_type=gatewayin
  gateway_real : xbsIndex_r4/Gateway In  gui_display_data_type=Fixed-point  arith_type="Signed  (2's comp)"  n_bits=18  bin_pt=17  preci_type=Single  exp_width=8  frac_width=24  quantization=Truncate  overflow=Wrap  period=1  dbl_ovrd=off  timing_constraint=None  locs_specified=off  LOCs={}  UseAsADC=off  ADCChannel='1'  inherit_from_input=off  hdl_port=on  block_type=gatewayin
  ri_to_c : Subsystem
  workspace_var : FromWorkspace  VariableName=X1  SampleTime=0
  X1 : Outport
  wires:
  ri_to_c/1(c) -> X1/1
  gateway_imag/1 -> ri_to_c/2(im)
  gateway_real/1 -> ri_to_c/1(re)
  c_to_ri_simulink/2 -> gateway_imag/1
  c_to_ri_simulink/1 -> gateway_real/1
  workspace_var/1 -> c_to_ri_simulink/1

== system kurtosis/multi_from_workspace_complex/from_workspace_cplx_2 ==
  c_to_ri_simulink : ComplexToRealImag
  gateway_imag : xbsIndex_r4/Gateway In  gui_display_data_type=Fixed-point  arith_type="Signed  (2's comp)"  n_bits=18  bin_pt=17  preci_type=Single  exp_width=8  frac_width=24  quantization=Truncate  overflow=Wrap  period=1  dbl_ovrd=off  timing_constraint=None  locs_specified=off  LOCs={}  UseAsADC=off  ADCChannel='1'  inherit_from_input=off  hdl_port=on  block_type=gatewayin
  gateway_real : xbsIndex_r4/Gateway In  gui_display_data_type=Fixed-point  arith_type="Signed  (2's comp)"  n_bits=18  bin_pt=17  preci_type=Single  exp_width=8  frac_width=24  quantization=Truncate  overflow=Wrap  period=1  dbl_ovrd=off  timing_constraint=None  locs_specified=off  LOCs={}  UseAsADC=off  ADCChannel='1'  inherit_from_input=off  hdl_port=on  block_type=gatewayin
  ri_to_c : Subsystem
  workspace_var : FromWorkspace  VariableName=X2  SampleTime=0
  X2 : Outport
  wires:
  ri_to_c/1(c) -> X2/1
  gateway_imag/1 -> ri_to_c/2(im)
  gateway_real/1 -> ri_to_c/1(re)
  c_to_ri_simulink/2 -> gateway_imag/1
  c_to_ri_simulink/1 -> gateway_real/1
  workspace_var/1 -> c_to_ri_simulink/1

== system kurtosis/multi_from_workspace_complex/from_workspace_cplx_3 ==
  c_to_ri_simulink : ComplexToRealImag
  gateway_imag : xbsIndex_r4/Gateway In  gui_display_data_type=Fixed-point  arith_type="Signed  (2's comp)"  n_bits=18  bin_pt=17  preci_type=Single  exp_width=8  frac_width=24  quantization=Truncate  overflow=Wrap  period=1  dbl_ovrd=off  timing_constraint=None  locs_specified=off  LOCs={}  UseAsADC=off  ADCChannel='1'  inherit_from_input=off  hdl_port=on  block_type=gatewayin
  gateway_real : xbsIndex_r4/Gateway In  gui_display_data_type=Fixed-point  arith_type="Signed  (2's comp)"  n_bits=18  bin_pt=17  preci_type=Single  exp_width=8  frac_width=24  quantization=Truncate  overflow=Wrap  period=1  dbl_ovrd=off  timing_constraint=None  locs_specified=off  LOCs={}  UseAsADC=off  ADCChannel='1'  inherit_from_input=off  hdl_port=on  block_type=gatewayin
  ri_to_c : Subsystem
  workspace_var : FromWorkspace  VariableName=X3  SampleTime=0
  X3 : Outport
  wires:
  ri_to_c/1(c) -> X3/1
  gateway_imag/1 -> ri_to_c/2(im)
  gateway_real/1 -> ri_to_c/1(re)
  c_to_ri_simulink/2 -> gateway_imag/1
  c_to_ri_simulink/1 -> gateway_real/1
  workspace_var/1 -> c_to_ri_simulink/1

== system kurtosis/multi_from_workspace_complex/from_workspace_cplx_4 ==
  c_to_ri_simulink : ComplexToRealImag
  gateway_imag : xbsIndex_r4/Gateway In  gui_display_data_type=Fixed-point  arith_type="Signed  (2's comp)"  n_bits=18  bin_pt=17  preci_type=Single  exp_width=8  frac_width=24  quantization=Truncate  overflow=Wrap  period=1  dbl_ovrd=off  timing_constraint=None  locs_specified=off  LOCs={}  UseAsADC=off  ADCChannel='1'  inherit_from_input=off  hdl_port=on  block_type=gatewayin
  gateway_real : xbsIndex_r4/Gateway In  gui_display_data_type=Fixed-point  arith_type="Signed  (2's comp)"  n_bits=18  bin_pt=17  preci_type=Single  exp_width=8  frac_width=24  quantization=Truncate  overflow=Wrap  period=1  dbl_ovrd=off  timing_constraint=None  locs_specified=off  LOCs={}  UseAsADC=off  ADCChannel='1'  inherit_from_input=off  hdl_port=on  block_type=gatewayin
  ri_to_c : Subsystem
  workspace_var : FromWorkspace  VariableName=X4  SampleTime=0
  X4 : Outport
  wires:
  ri_to_c/1(c) -> X4/1
  gateway_imag/1 -> ri_to_c/2(im)
  gateway_real/1 -> ri_to_c/1(re)
  c_to_ri_simulink/2 -> gateway_imag/1
  c_to_ri_simulink/1 -> gateway_real/1
  workspace_var/1 -> c_to_ri_simulink/1

== system kurtosis/multi_from_workspace_complex/from_workspace_cplx_5 ==
  c_to_ri_simulink : ComplexToRealImag
  gateway_imag : xbsIndex_r4/Gateway In  gui_display_data_type=Fixed-point  arith_type="Signed  (2's comp)"  n_bits=18  bin_pt=17  preci_type=Single  exp_width=8  frac_width=24  quantization=Truncate  overflow=Wrap  period=1  dbl_ovrd=off  timing_constraint=None  locs_specified=off  LOCs={}  UseAsADC=off  ADCChannel='1'  inherit_from_input=off  hdl_port=on  block_type=gatewayin
  gateway_real : xbsIndex_r4/Gateway In  gui_display_data_type=Fixed-point  arith_type="Signed  (2's comp)"  n_bits=18  bin_pt=17  preci_type=Single  exp_width=8  frac_width=24  quantization=Truncate  overflow=Wrap  period=1  dbl_ovrd=off  timing_constraint=None  locs_specified=off  LOCs={}  UseAsADC=off  ADCChannel='1'  inherit_from_input=off  hdl_port=on  block_type=gatewayin
  ri_to_c : Subsystem
  workspace_var : FromWorkspace  VariableName=X5  SampleTime=0
  X5 : Outport
  wires:
  ri_to_c/1(c) -> X5/1
  gateway_imag/1 -> ri_to_c/2(im)
  gateway_real/1 -> ri_to_c/1(re)
  c_to_ri_simulink/2 -> gateway_imag/1
  c_to_ri_simulink/1 -> gateway_real/1
  workspace_var/1 -> c_to_ri_simulink/1

== system kurtosis/multi_from_workspace_complex/from_workspace_cplx_6 ==
  c_to_ri_simulink : ComplexToRealImag
  gateway_imag : xbsIndex_r4/Gateway In  gui_display_data_type=Fixed-point  arith_type="Signed  (2's comp)"  n_bits=18  bin_pt=17  preci_type=Single  exp_width=8  frac_width=24  quantization=Truncate  overflow=Wrap  period=1  dbl_ovrd=off  timing_constraint=None  locs_specified=off  LOCs={}  UseAsADC=off  ADCChannel='1'  inherit_from_input=off  hdl_port=on  block_type=gatewayin
  gateway_real : xbsIndex_r4/Gateway In  gui_display_data_type=Fixed-point  arith_type="Signed  (2's comp)"  n_bits=18  bin_pt=17  preci_type=Single  exp_width=8  frac_width=24  quantization=Truncate  overflow=Wrap  period=1  dbl_ovrd=off  timing_constraint=None  locs_specified=off  LOCs={}  UseAsADC=off  ADCChannel='1'  inherit_from_input=off  hdl_port=on  block_type=gatewayin
  ri_to_c : Subsystem
  workspace_var : FromWorkspace  VariableName=X6  SampleTime=0
  X6 : Outport
  wires:
  ri_to_c/1(c) -> X6/1
  gateway_imag/1 -> ri_to_c/2(im)
  gateway_real/1 -> ri_to_c/1(re)
  c_to_ri_simulink/2 -> gateway_imag/1
  c_to_ri_simulink/1 -> gateway_real/1
  workspace_var/1 -> c_to_ri_simulink/1

== system kurtosis/multi_from_workspace_complex/from_workspace_cplx_7 ==
  c_to_ri_simulink : ComplexToRealImag
  gateway_imag : xbsIndex_r4/Gateway In  gui_display_data_type=Fixed-point  arith_type="Signed  (2's comp)"  n_bits=18  bin_pt=17  preci_type=Single  exp_width=8  frac_width=24  quantization=Truncate  overflow=Wrap  period=1  dbl_ovrd=off  timing_constraint=None  locs_specified=off  LOCs={}  UseAsADC=off  ADCChannel='1'  inherit_from_input=off  hdl_port=on  block_type=gatewayin
  gateway_real : xbsIndex_r4/Gateway In  gui_display_data_type=Fixed-point  arith_type="Signed  (2's comp)"  n_bits=18  bin_pt=17  preci_type=Single  exp_width=8  frac_width=24  quantization=Truncate  overflow=Wrap  period=1  dbl_ovrd=off  timing_constraint=None  locs_specified=off  LOCs={}  UseAsADC=off  ADCChannel='1'  inherit_from_input=off  hdl_port=on  block_type=gatewayin
  ri_to_c : Subsystem
  workspace_var : FromWorkspace  VariableName=X7  SampleTime=0
  X7 : Outport
  wires:
  ri_to_c/1(c) -> X7/1
  gateway_imag/1 -> ri_to_c/2(im)
  gateway_real/1 -> ri_to_c/1(re)
  c_to_ri_simulink/2 -> gateway_imag/1
  c_to_ri_simulink/1 -> gateway_real/1
  workspace_var/1 -> c_to_ri_simulink/1

== system kurtosis/multi_from_workspace_complex/from_workspace_cplx_8 ==
  c_to_ri_simulink : ComplexToRealImag
  gateway_imag : xbsIndex_r4/Gateway In  gui_display_data_type=Fixed-point  arith_type="Signed  (2's comp)"  n_bits=18  bin_pt=17  preci_type=Single  exp_width=8  frac_width=24  quantization=Truncate  overflow=Wrap  period=1  dbl_ovrd=off  timing_constraint=None  locs_specified=off  LOCs={}  UseAsADC=off  ADCChannel='1'  inherit_from_input=off  hdl_port=on  block_type=gatewayin
  gateway_real : xbsIndex_r4/Gateway In  gui_display_data_type=Fixed-point  arith_type="Signed  (2's comp)"  n_bits=18  bin_pt=17  preci_type=Single  exp_width=8  frac_width=24  quantization=Truncate  overflow=Wrap  period=1  dbl_ovrd=off  timing_constraint=None  locs_specified=off  LOCs={}  UseAsADC=off  ADCChannel='1'  inherit_from_input=off  hdl_port=on  block_type=gatewayin
  ri_to_c : Subsystem
  workspace_var : FromWorkspace  VariableName=X8  SampleTime=0
  X8 : Outport
  wires:
  ri_to_c/1(c) -> X8/1
  gateway_imag/1 -> ri_to_c/2(im)
  gateway_real/1 -> ri_to_c/1(re)
  c_to_ri_simulink/2 -> gateway_imag/1
  c_to_ri_simulink/1 -> gateway_real/1
  workspace_var/1 -> c_to_ri_simulink/1

== system kurtosis/multi_to_workspace_complex/to_workspace_cplx_1 ==
  X_fi1 : Inport
  c_to_ri : Subsystem
  imag_gateway : xbsIndex_r4/Gateway Out  inherit_from_input=on  hdl_port=off  timing_constraint=None  locs_specified=off  LOCs={}  UseAsDAC=off  DACChannel='1'  block_type=gatewayout
  real_gateway : xbsIndex_r4/Gateway Out  inherit_from_input=on  hdl_port=off  timing_constraint=None  locs_specified=off  LOCs={}  UseAsDAC=off  DACChannel='1'  block_type=gatewayout
  ri_to_c : RealImagToComplex
  workspace_output : ToWorkspace  VariableName=X_fi1  SampleTime=-1
  _o : Outport
  wires:
  X_fi1/1 -> c_to_ri/1(c), _o/1
  ri_to_c/1 -> workspace_output/1  "cplx"
  imag_gateway/1 -> ri_to_c/2
  real_gateway/1 -> ri_to_c/1
  c_to_ri/2(im) -> imag_gateway/1  "c_to_ri_out2"
  c_to_ri/1(re) -> real_gateway/1  "c_to_ri_out1"
